simulink model "LaneKeeping"  (R2022b)
settings: Solver=ode8  StartTime=0.0  StopTime=inf  FixedStep=0.001  RelTol=1e-3
InitFcn:
  | start = 1
StopFcn:
  | start = 0
model workspace (MAT data in the model file):
  SL_ROS_VariableLengthArrays_MaxSizes.CommonInfo.ArrayTruncateAction = 'EmitWarning'
  SL_ROS_VariableLengthArrays_MaxSizes.MsgTypeMap = containers.Map
  SL_ROS_VariableLengthArrays_MaxSizes.MsgTypeMap.serialization.keys = {'sensor_msgs/CompressedImage'}
  SL_ROS_VariableLengthArrays_MaxSizes.MsgTypeMap.serialization.values{1}(1).PropertyName = 'Data'
  SL_ROS_VariableLengthArrays_MaxSizes.MsgTypeMap.serialization.values{1}(1).DataType = 'uint8'
  SL_ROS_VariableLengthArrays_MaxSizes.MsgTypeMap.serialization.values{1}(1).MaxLength = 220631000
  SL_ROS_VariableLengthArrays_MaxSizes.MsgTypeMap.serialization.values{1}(2).PropertyName = 'Format'
  SL_ROS_VariableLengthArrays_MaxSizes.MsgTypeMap.serialization.values{1}(2).DataType = 'uint8'
  SL_ROS_VariableLengthArrays_MaxSizes.MsgTypeMap.serialization.values{1}(2).MaxLength = 128
  SL_ROS_VariableLengthArrays_MaxSizes.MsgTypeMap.serialization.uniformity = 0
  SL_ROS_VariableLengthArrays_MaxSizes.MsgTypeMap.serialization.keyType = 'char'
  SL_ROS_VariableLengthArrays_MaxSizes.MsgTypeMap.serialization.valueType = 'any'
undefined symbols (not defined in the file): gray, L, r, Rec, SDTV, VelLeft, VelRight
libraries: robotlib x6, visiontextngfix x6, simulink_extras x6, visionconversions x5, visiontransforms x4, dspstat3 x4, dspmtrx3 x4, visionfilter x2, matrix_library x2, visionanalysis x2, visionstatistics x2, slpidlib x1
settings Model: Creator=gaetano  LastModifiedBy=gaetano

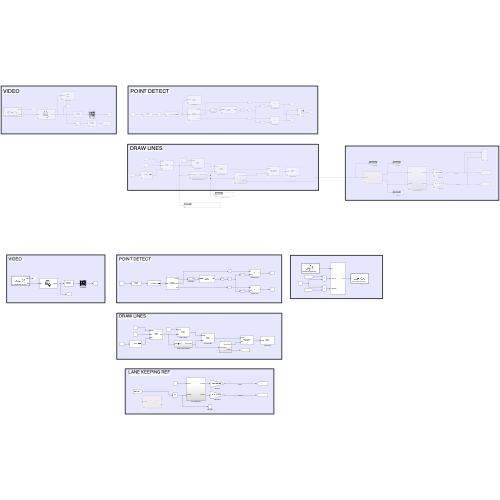
[thumbnail: Simulink's stored preview of the top-level diagram]
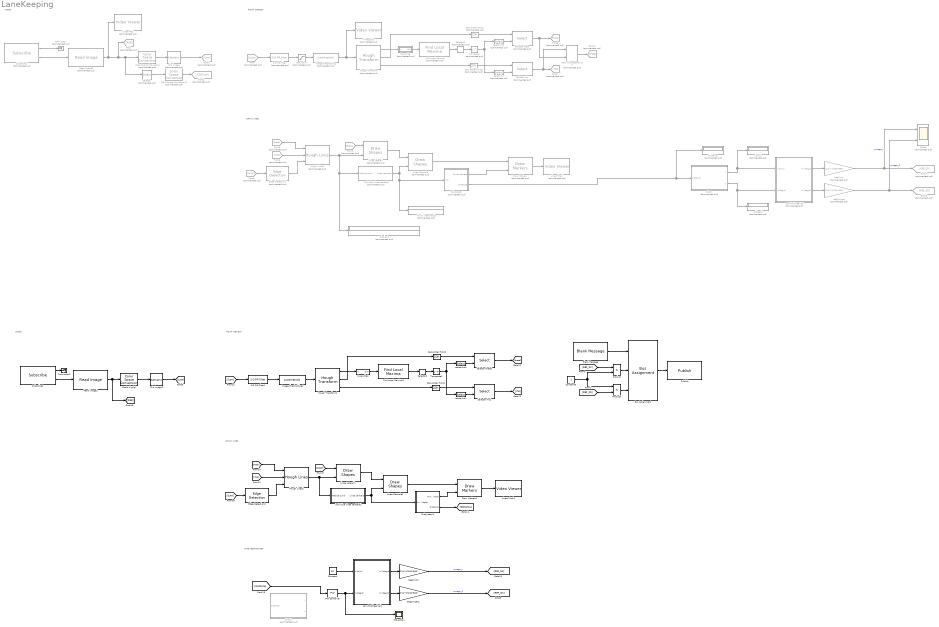
== system LaneKeeping ==
  note: VIDEO
  note: POINT DETECT
  note: DRAW LINES
  note: LANE KEEPING REF
  note: DRAW LINES
  note: POINT DETECT
  note: VIDEO
  2-D FIR Filter : visionfilter/2-D FIR Filter  Commented=on  separable=off  filtSrc=Specify via dialog  filterMtrx=[-1 0 1]  verticalFilter=[4 0]  horizontalFilter=[4 0]  outSize=Same as input port I  padType=Replicate  padSrc=Specify via dialog  padVal=0  method=Convolution  firstCoeffMode=Specify word length  firstCoeffWordLength=16  firstCoeffFracLength=14  firstCoeffSignedness=Signed  firstCoeffLastDataTypeStr=fixdt(1,16)  outputSignedness=Auto  accumLastDataTypeStr=Inherit: Same as product output  prodOutputMode=Binary point scaling  prodOutputWordLength=32  prodOutputFracLength=10  prodOutputLastDataTypeStr=fixdt([],32,10)  roundingMode=Floor  overflowMode=on  firstCoeffDataTypeStr=fixdt(1,16)  firstCoeffMin=[]  firstCoeffMax=[]  prodOutputDataTypeStr=fixdt([],32,10)  accumDataTypeStr=Inherit: Same as product output  outputMin=[]  outputMax=[]
  2-D FIR Filter1 : visionfilter/2-D FIR Filter  separable=off  filtSrc=Specify via dialog  filterMtrx=[-1 0 1]  verticalFilter=[4 0]  horizontalFilter=[4 0]  outSize=Same as input port I  padType=Replicate  padSrc=Specify via dialog  padVal=0  method=Convolution  firstCoeffMode=Specify word length  firstCoeffWordLength=16  firstCoeffFracLength=14  firstCoeffSignedness=Signed  firstCoeffLastDataTypeStr=fixdt(1,16)  outputSignedness=Auto  accumLastDataTypeStr=Inherit: Same as product output  prodOutputMode=Binary point scaling  prodOutputWordLength=32  prodOutputFracLength=10  prodOutputLastDataTypeStr=fixdt([],32,10)  roundingMode=Floor  overflowMode=on  firstCoeffDataTypeStr=fixdt(1,16)  firstCoeffMin=[]  firstCoeffMax=[]  prodOutputDataTypeStr=fixdt([],32,10)  accumDataTypeStr=Inherit: Same as product output  outputMin=[]  outputMax=[]
  Blank Message : robotlib/Blank Message  messageClass=Message  entityType=duckietown_msgs/WheelsCmdStamped  messageType=duckietown_msgs/WheelsCmdStamped  SampleTime=-1  legacyBusStruct=off
      settings: LibrarySourceBlock=roslib/ROS/Blank Message
  Bus Assignment : BusAssignment  AssignedSignals=VelLeft,VelRight
  Chart : Stateflow chart  Commented=on  TreatAsAtomicUnit=on
  Chart1 : Stateflow chart  Commented=on  TreatAsAtomicUnit=on
  Clip image : matrix_library/Submatrix  Commented=on  RowSpan=Range of rows  RowStartMode=Offset from middle  RowStartIndex=1  RowEndMode=Last  RowEndIndex=1  ColSpan=All columns  ColStartMode=First  ColStartIndex=1  ColEndMode=Last  ColEndIndex=1
  Clip image1 : matrix_library/Submatrix  RowSpan=Range of rows  RowStartMode=Offset from middle  RowStartIndex=15  RowEndMode=Last  RowEndIndex=1  ColSpan=All columns  ColStartMode=First  ColStartIndex=1  ColEndMode=Last  ColEndIndex=1
  Color Space Conversion : visionconversions/Color Space  Conversion  Commented=on  conversion=Obsolete  conversionActive=R'G'B' to intensity  wp_str=D65  rec=Rec. 601 (SDTV)  sys=1125/60/2:1  imagePorts=One multidimensional signal
  Color Space Conversion1 : visionconversions/Color Space  Conversion  Commented=on  conversion=Obsolete  conversionActive=R'G'B' to Y'CbCr  wp_str=D65  rec=Rec. 601 (SDTV)  sys=1125/60/2:1  imagePorts=One multidimensional signal
  Constant : Constant  Value=10
  Constant3 : Constant  OutDataTypeStr=single
  Display2 : Display  Commented=on
  Distanza : Display  Commented=on
  Draw Markers : visiontextngfix/Draw Markers  Commented=on  shape=X-mark  size=3  fill=off  fillClrSource=Specify via dialog  display=White  intensity=200  color=[250 0 0]  opacity=0.6  viewport=Entire image  antialiasing=off  inType=Obsolete  imagePorts=One multidimensional signal  roundingMode=Floor  overflowMode=off  memoryMode=Specify word length  memoryWordLength=16  memoryFracLength=15  prodOutputMode=Binary point scaling  prodOutputWordLength=32  prodOutputFracLength=14
  Draw Markers1 : visiontextngfix/Draw Markers  shape=X-mark  size=3  fill=off  fillClrSource=Specify via dialog  display=White  intensity=200  color=[250 0 0]  opacity=0.6  viewport=Entire image  antialiasing=off  inType=Obsolete  imagePorts=One multidimensional signal  roundingMode=Floor  overflowMode=off  memoryMode=Specify word length  memoryWordLength=16  memoryFracLength=15  prodOutputMode=Binary point scaling  prodOutputWordLength=32  prodOutputFracLength=14
  Edge Detection1 : visionanalysis/Edge Detection  Commented=on  method=Sobel  outputType=Binary image  userDefinedThreshold=off  thresholdSource=Input port  threshold=20  thresholdTuning=4  edgeThinning=off  threshold_canny=[0.25 0.60]  autoPercent=70  sigma=1  roundingMode=Floor  overflowMode=off  prodOutputMode=Binary point scaling  prodOutputWordLength=32  prodOutputFracLength=8
  Edge Detection2 : visionanalysis/Edge Detection  method=Sobel  outputType=Binary image  userDefinedThreshold=off  thresholdSource=Input port  threshold=20  thresholdTuning=4  edgeThinning=off  threshold_canny=[0.25 0.60]  autoPercent=70  sigma=1  roundingMode=Floor  overflowMode=off  prodOutputMode=Binary point scaling  prodOutputWordLength=32  prodOutputFracLength=8
  Find Local Maxima : visionstatistics/Find Local Maxima  Commented=on  num_peaks=2  nhood_size=[301 81]  src_thresh=Obsolete9b  src_thresh_inuse=Specify via dialog  threshold=1  inputIsHough=on  dt_peak=uint16  isOutVarDim=on  dt_count=uint16
  Find Local Maxima1 : visionstatistics/Find Local Maxima  num_peaks=2  nhood_size=[301 81]  src_thresh=Obsolete9b  src_thresh_inuse=Specify via dialog  threshold=1  inputIsHough=on  dt_peak=uint16  isOutVarDim=on  dt_count=uint16
  From : From  Commented=on  GotoTag=ILow
  From5 : From  Commented=on  GotoTag=theta
  From6 : From  Commented=on  GotoTag=rho
  From8 : From  Commented=on  GotoTag=ILow
  From9 : From  Commented=on  GotoTag=ILow
  Goto : Goto  Commented=on  GotoTag=RGB
  Goto1 : Goto  Commented=on  GotoTag=ILow
  Goto2 : Goto  Commented=on  GotoTag=YCbCrLow
  Goto3 : Goto  Commented=on  GotoTag=REF_DX
  Goto4 : Goto  Commented=on  GotoTag=REF_SX
  Goto6 : Goto  Commented=on  GotoTag=theta
  Goto7 : Goto  Commented=on  GotoTag=rho
  Goto8 : Goto  Commented=on  GotoTag=lines
  Hough Lines1 : visiontransforms/Hough Lines  Commented=on  sineCompMethod=Trigonometric function  thetaRes=pi/180  roundingMode=Nearest  overflowMode=on  firstCoeffMode=Specify word length  firstCoeffWordLength=16  prodOutputMode=Binary point scaling  prodOutputWordLength=32  prodOutputFracLength=16  firstCoeffFracLength=15
  Hough Lines2 : visiontransforms/Hough Lines  sineCompMethod=Trigonometric function  thetaRes=pi/180  roundingMode=Nearest  overflowMode=on  firstCoeffMode=Specify word length  firstCoeffWordLength=16  prodOutputMode=Binary point scaling  prodOutputWordLength=32  prodOutputFracLength=16  firstCoeffFracLength=15
  Hough Transform : visiontransforms/Hough Transform  Commented=on  theta_res=pi/180  rho_res=1  out_theta_rho=on  outdtmode=single  roundingMode=Nearest  overflowMode=on  firstCoeffMode=Binary point scaling  firstCoeffWordLength=16  firstCoeffFracLength=14  secondCoeffMode=Binary point scaling  secondCoeffWordLength=32  secondCoeffFracLength=16  prodOutputMode=Binary point scaling  prodOutputWordLength=32  prodOutputFracLength=20  accumMode=Binary point scaling  accumWordLength=32  accumFracLength=20  outputMode=Binary point scaling  outputWordLength=16  outputFracLength=0  memoryMode=Binary point scaling  memoryWordLength=32  memoryFracLength=16
  Hough Transform1 : visiontransforms/Hough Transform  theta_res=pi/180  rho_res=1  out_theta_rho=on  outdtmode=single  roundingMode=Nearest  overflowMode=on  firstCoeffMode=Binary point scaling  firstCoeffWordLength=16  firstCoeffFracLength=14  secondCoeffMode=Binary point scaling  secondCoeffWordLength=32  secondCoeffFracLength=16  prodOutputMode=Binary point scaling  prodOutputWordLength=32  prodOutputFracLength=20  accumMode=Binary point scaling  accumWordLength=32  accumFracLength=20  outputMode=Binary point scaling  outputWordLength=16  outputFracLength=0  memoryMode=Binary point scaling  memoryWordLength=32  memoryFracLength=16
  Image thresholding : visionconversions/Autothreshold  Commented=on  operator=>  threshOut=off  effMetricOut=off  userDefinedRange=off  umin=50  umax=255  outOfRngOpt=Ignore  scaleThreshold=off  scaleFactor=1  roundingMode=Floor  overflowMode=off  P1Mode=Specify word length  P1WordLength=32  P1FracLength=30  P2Mode=Specify word length  P2WordLength=32  P2FracLength=22  P3Mode=Specify word length  P3WordLength=32  P3FracLength=14  P4Mode=Binary point scaling  P4WordLength=32  P4FracLength=15  Q1Mode=Specify word length  Q1WordLength=32  Q1FracLength=16  EMMode=Specify word length  EMWordLength=16  EMFracLength=14
  Image thresholding1 : visionconversions/Autothreshold  operator=>  threshOut=off  effMetricOut=off  userDefinedRange=off  umin=50  umax=255  outOfRngOpt=Ignore  scaleThreshold=off  scaleFactor=1  roundingMode=Floor  overflowMode=off  P1Mode=Specify word length  P1WordLength=32  P1FracLength=30  P2Mode=Specify word length  P2WordLength=32  P2FracLength=22  P3Mode=Specify word length  P3WordLength=32  P3FracLength=14  P4Mode=Binary point scaling  P4WordLength=32  P4FracLength=15  Q1Mode=Specify word length  Q1WordLength=32  Q1FracLength=16  EMMode=Specify word length  EMWordLength=16  EMFracLength=14
  Individua linea centrale : Subsystem  Commented=on
  Individua linea centrale1 : Subsystem
  Linea Centrale : visiontextngfix/Draw Shapes  Commented=on  shape=Lines  fill=off  lineWidth=2  fillClrSource=Specify via dialog  display=White  intensity=200  color=[200 255 100]  opacity=0.6  viewport=Entire image  antialiasing=off  inType=Obsolete  imagePorts=One multidimensional signal  roundingMode=Floor  overflowMode=off  memoryMode=Specify word length  memoryWordLength=16  prodOutputMode=Binary point scaling  prodOutputWordLength=32  prodOutputFracLength=14  memoryFracLength=15
  Linea Centrale1 : visiontextngfix/Draw Shapes  shape=Lines  fill=off  lineWidth=2  fillClrSource=Specify via dialog  display=White  intensity=200  color=[200 255 100]  opacity=0.6  viewport=Entire image  antialiasing=off  inType=Obsolete  imagePorts=One multidimensional signal  roundingMode=Floor  overflowMode=off  memoryMode=Specify word length  memoryWordLength=16  prodOutputMode=Binary point scaling  prodOutputWordLength=32  prodOutputFracLength=14  memoryFracLength=15
  Linee Finali : VideoViewer  Commented=on  colormapValue=gray(256)  FigPos=[831 826 610 698]
  Linee Finali1 : VideoViewer  colormapValue=gray(256)  FigPos=[342 823 793 695]
  Linee Laterali : visiontextngfix/Draw Shapes  Commented=on  shape=Lines  fill=off  lineWidth=2  fillClrSource=Specify via dialog  display=White  intensity=200  color=[200 255 100]  opacity=0.6  viewport=Entire image  antialiasing=off  inType=Obsolete  imagePorts=One multidimensional signal  roundingMode=Floor  overflowMode=off  memoryMode=Specify word length  memoryWordLength=16  prodOutputMode=Binary point scaling  prodOutputWordLength=32  prodOutputFracLength=14  memoryFracLength=15
  Linee Laterali1 : visiontextngfix/Draw Shapes  shape=Lines  fill=off  lineWidth=2  fillClrSource=Specify via dialog  display=White  intensity=200  color=[200 255 100]  opacity=0.6  viewport=Entire image  antialiasing=off  inType=Obsolete  imagePorts=One multidimensional signal  roundingMode=Floor  overflowMode=off  memoryMode=Specify word length  memoryWordLength=16  prodOutputMode=Binary point scaling  prodOutputWordLength=32  prodOutputFracLength=14  memoryFracLength=15
  Matrix Concatenation3 : Concatenate  Commented=on  Mode=Multidimensional array
  Overwrite : Subsystem  Commented=on
  Overwrite1 : Subsystem
  PID Controller : slpidlib/PID Controller  Controller=P  Form=Parallel  TimeDomain=Continuous-time  UseExternalTs=off  SampleTime=-1  IntegratorMethod=Forward Euler  FilterMethod=Forward Euler  ControllerParametersSource=internal  P=0.28  I=1  UseKiTs=off  D=0  N=100  UseFilter=on  TunerSelectOption=Transfer Function Based (PID Tuner App)  InitialConditionSource=internal  InitialConditionForIntegrator=0  InitialConditionForFilter=0  DifferentiatorICPrevScaledInput=0  ExternalReset=none  TrackingMode=off  Kt=1  LimitOutput=off  SatLimitsSource=internal  UpperSaturationLimit=40  LowerSaturationLimit=-40  LinearizeAsGain=off  AntiWindupMode=none  Kb=1  LimitIntegrator=off  UpperIntegratorSaturationLimit=inf  LowerIntegratorSaturationLimit=-inf  PGainOutDataTypeStr=double  PProdOutDataTypeStr=double  POutMin=[]  POutMax=[]  IOutMin=[]  IOutMax=[]  DOutMin=[]  DOutMax=[]  NOutMin=[]  NOutMax=[]  SumOutMin=[]  SumOutMax=[]  SaturationOutMin=[]  SaturationOutMax=[]  PParamMin=[]  PParamMax=[]  IParamMin=[]  IParamMax=[]  DParamMin=[]  DParamMax=[]  NParamMin=[]  NParamMax=[]  KbParamMin=[]  KbParamMax=[]  KtParamMin=[]  KtParamMax=[]  KbOutMin=[]  KbOutMax=[]  KtOutMin=[]  KtOutMax=[]  IntegratorOutMin=[]  IntegratorOutMax=[]  FilterOutMin=[]  FilterOutMax=[]  SumI1OutMin=[]  SumI1OutMax=[]  SumI2OutMin=[]  SumI2OutMax=[]  SumI3OutMin=[]  SumI3OutMax=[]  SumI4OutMin=[]  SumI4OutMax=[]  SumDOutMin=[]  SumDOutMax=[]  DifferentiatorOutMin=[]  DifferentiatorOutMax=[]  FilterDiffOutCoefMin=[]  FilterDiffOutCoefMax=[]  ReciprocalOutMin=[]  ReciprocalOutMax=[]  SumDenOutMin=[]  SumDenOutMax=[]  SumNumOutMin=[]  SumNumOutMax=[]  DivideOutMin=[]  DivideOutMax=[]  UdiffTsProdOutMin=[]  UdiffTsProdOutMax=[]  NTsProdOutMin=[]  NTsProdOutMax=[]  UintegralTsProdOutMin=[]  UintegralTsProdOutMax=[]  UngainTsProdOutMin=[]  UngainTsProdOutMax=[]  ClampingZeroOutDataTypeStr=Inherit: Inherit via back propagation  ClampingZeroOutMin=[]  ClampingZeroOutMax=[]  FilterDenConstantOutDataTypeStr=Inherit: Inherit via back propagation  FilterDenConstantOutMin=[]  FilterDenConstantOutMax=[]  PCopyOutDataTypeStr=Inherit: Inherit via back propagation  PCopyOutMin=[]  PCopyOutMax=[]  NCopyOutDataTypeStr=Inherit: Inherit via back propagation  NCopyOutMin=[]  NCopyOutMax=[]  IntegratorContinuousStateAttributes=''  IntegratorStateMustResolveToSignalObject=off  IntegratorRTWStateStorageClass=Auto  FilterContinuousStateAttributes=''  FilterStateMustResolveToSignalObject=off  FilterRTWStateStorageClass=Auto  ParallelPVariant=InternalParameters  IdealPVariant=Disabled  IVariant=Disabled  DVariant=Disabled  IntegratorVariant=Disabled  SatVariant=Disabled  AWVariant=Disabled  PCopyVariant=Disabled  TRVariant=Disabled  FdbkBlocksVariant=Forward  IdealPFdbkVariant=Disabled  SatFdbkVariant=Disabled  DerivativeFilterVariant=Disabled  NVariant=Disabled  NCopyVariant=Disabled_SignalSpec  FilterICVariant=Disabled  IntegratorICVariant=Disabled  ExternalResetVariant=Disabled  TRSumVariant=Passthrough  SumFdbkVariant=Disabled  SumVariant=Passthrough_P  TsampFilterVariant=InternalTs  TsampNgainVariant=Passthrough  TsampIntegralVariant=Disabled_SignalSpec  ExternalSaturationOutDataTypeStr=Inherit: Same as second input
  PID_action : Scope
  Product : Product  OutDataTypeStr=single
  Product1 : Product  OutDataTypeStr=single
  Publish : robotlib/Publish  topicSource=Select from ROS network  topic=/vic9osimhen/wheels_driver_node/wheels_cmd  messageType=duckietown_msgs/WheelsCmdStamped  legacyBusStruct=off  messageQueueLength=1
      settings: LibrarySourceBlock=roslib/ROS/Publish
  Punti linea media : Display  Commented=on
  Read Image1 : robotlib/Read Image  Commented=on  MaximumImageSize=[480,640]  ImageEncoding=rgb8  ShowAlphaOutput=off  ShowErrorCodeOutput=off  VariableSizeOutputs=off
      settings: LibrarySourceBlock=roslib/ROS/Read Image
  Read Image2 : robotlib/Read Image  MaximumImageSize=[480,640]  ImageEncoding=rgb8  ShowAlphaOutput=off  ShowErrorCodeOutput=off  VariableSizeOutputs=off
      settings: LibrarySourceBlock=roslib/ROS/Read Image
  Saturation : Saturate  Commented=on  UpperLimit=1  LowerLimit=0
  Scala di grigi : visionconversions/Color Space  Conversion  conversion=Obsolete  conversionActive=R'G'B' to intensity  wp_str=D65  rec=Rec. 601 (SDTV)  sys=1125/60/2:1  imagePorts=One multidimensional signal
  Scope : Scope  Commented=on  NumInputPorts=2
  Selector : Selector  Commented=on  NumberOfDimensions=3  InputPortWidth=3  IndexOptions=Index vector (dialog),Select all,Select all  Indices=(640/2+1):480,1,2  OutputSizes=1,1,1
  Selector rho : Selector  Commented=on  NumberOfDimensions=2  InputPortWidth=3  IndexOptions=Select all,Index vector (port)  Indices=1,2  OutputSizes=1,1
  Selector rho1 : Selector  NumberOfDimensions=2  InputPortWidth=3  IndexOptions=Select all,Index vector (port)  Indices=1,2  OutputSizes=1,1
  Selector theta : Selector  Commented=on  NumberOfDimensions=2  InputPortWidth=3  IndexOptions=Select all,Index vector (port)  Indices=1,2  OutputSizes=1,1
  Selector theta1 : Selector  NumberOfDimensions=2  InputPortWidth=3  IndexOptions=Select all,Index vector (port)  Indices=1,2  OutputSizes=1,1
  Selector1 : Selector  Commented=on  NumberOfDimensions=2  InputPortWidth=3  IndexOptions=Select all,Index vector (dialog)  Indices=[2 1],[2 1]  OutputSizes=1,1
  Selector2 : Selector  NumberOfDimensions=2  InputPortWidth=3  IndexOptions=Select all,Index vector (dialog)  Indices=[2 1],[2 1]  OutputSizes=1,1
  Subscribe1 : robotlib/Subscribe  Commented=on  topicSource=Select from ROS network  topic=/vic9osimhen/camera_node/image/compressed  messageType=sensor_msgs/CompressedImage  SampleTime=-1  legacyBusStruct=off  messageQueueLength=1
      settings: LibrarySourceBlock=roslib/ROS/Subscribe
  Subscribe2 : robotlib/Subscribe  topicSource=Select from ROS network  topic=/vic9osimhen/camera_node/image/compressed  messageType=sensor_msgs/CompressedImage  SampleTime=-1  legacyBusStruct=off  messageQueueLength=1
      settings: LibrarySourceBlock=roslib/ROS/Subscribe
  Subsystem : Subsystem  Commented=on
  Subsystem1 : Subsystem
  Terminator : Terminator  Commented=on
  Terminator1 : Terminator
  Threshold : VideoViewer  Commented=on  colormapValue=gray(256)  FigPos=[280 584 557 295]
  Transpose : Math  Commented=on  Operator=transpose  SignedPower=on
  Transpose1 : Math  Operator=transpose  SignedPower=on
  Video ROS : VideoViewer  Commented=on  colormapValue=gray(256)  FigPos=[1 826 566 334]
  Zero-Order Hold1 : ZeroOrderHold  Commented=on  SampleTime=-1
  Zero-Order Hold2 : ZeroOrderHold  SampleTime=-1
  Zero-Order Hold3 : ZeroOrderHold  Commented=on  SampleTime=-1
  Zero-Order Hold4 : ZeroOrderHold  SampleTime=-1
  convToWheelVel : Subsystem  Commented=on
  convToWheelVel1 : Subsystem
  deg2m/s : Gain  Commented=on  Gain=(2*pi*r)/(100*360)
  deg2m/s1 : Gain  Gain=(2*pi*r)/(100*360)
  deg2m/sec : Gain  Commented=on  Gain=(2*pi*r)/(100*360)
  deg2m/sec1 : Gain  Gain=(2*pi*r)/(100*360)
  select rho : Selector  Commented=on  NumberOfDimensions=2  InputPortWidth=3  IndexOptions=Index vector (dialog),Select all  Indices=1,-1  OutputSizes=1
  select rho1 : Selector  NumberOfDimensions=2  InputPortWidth=3  IndexOptions=Index vector (dialog),Select all  Indices=1,-1  OutputSizes=1
  select rho2 : Selector  NumberOfDimensions=2  InputPortWidth=3  IndexOptions=Index vector (dialog),Select all  Indices=2,-1  OutputSizes=1
  select rho3 : Selector  Commented=on  NumberOfDimensions=2  InputPortWidth=3  IndexOptions=Index vector (dialog),Select all  Indices=2,-1  OutputSizes=1
  v(cm/s) : Display  Commented=on
  w(deg/s) : Display  Commented=on
  wires:
  Color Space Conversion/1 -> Clip image/1
  Color Space Conversion1/1 -> Goto2/1
  Clip image/1 -> Goto1/1
  Selector/1 -> Color Space Conversion1/1
  From/1 -> 2-D FIR Filter/1
  Image thresholding/1 -> Hough Transform/1, Threshold/1
  2-D FIR Filter/1 -> Saturation/1
  Saturation/1 -> Image thresholding/1
  Matrix Concatenation3/1 -> Goto8/1
  Hough Transform/1 -> Overwrite/1(In)
  Transpose/1 -> select rho/1, select rho3/1
  Selector1/1 -> Transpose/1
  Find Local Maxima/1 -> Selector1/1
  Hough Transform/3 -> Zero-Order Hold3/1
  select rho/1 -> Selector rho/2
  Zero-Order Hold3/1 -> Selector rho/1
  Hough Transform/2 -> Zero-Order Hold1/1
  select rho3/1 -> Selector theta/2
  Zero-Order Hold1/1 -> Selector theta/1
  Selector rho/1 -> Goto7/1, Matrix Concatenation3/1
  Selector theta/1 -> Goto6/1, Matrix Concatenation3/2
  Overwrite/1(Out) -> Find Local Maxima/1
  From5/1 -> Hough Lines1/1
  Edge Detection1/1 -> Hough Lines1/3
  From6/1 -> Hough Lines1/2
  Subscribe1/1 -> Terminator/1
  Subscribe1/2 -> Read Image1/1
  From8/1 -> Edge Detection1/1
  From9/1 -> Linee Laterali/1
  Linee Laterali/1 -> Linea Centrale/1
  Linea Centrale/1 -> Draw Markers/1
  Hough Lines1/1 -> Display2/1, Individua linea centrale/1(Matrice punti), Linee Laterali/2
  Individua linea centrale/1(Linea centrale) -> Linea Centrale/2, Punti linea media/1, Subsystem/1(In1)
  Draw Markers/1 -> Linee Finali/1
  Subsystem/1(Punto camera) -> Draw Markers/2
  Subsystem/2(Distanza) -> Distanza/1, Chart/1(distanza)
  Chart/1(v) -> v(cm/s)/1, convToWheelVel/1(v(cm/s))
  Chart/2(w) -> convToWheelVel/2(w(deg/s)), w(deg/s)/1
  convToWheelVel/1(wl (deg/s)) -> deg2m/s/1
  deg2m/sec/1 -> Goto3/1, Scope/2  "omega_R"
  deg2m/s/1 -> Goto4/1, Scope/1  "omega_L"
  convToWheelVel/2(wr (deg/s)) -> deg2m/sec/1
  Bus Assignment/1 -> Publish/1
  Blank Message/1 -> Bus Assignment/1
  Product/1 -> Bus Assignment/2
  Product1/1 -> Bus Assignment/3
  [REF_SX] -> Product/1
  [REF_DX] -> Product1/2
  Constant3/1 -> Product1/1, Product/2
  Read Image1/1 -> Color Space Conversion/1, Selector/1, Goto/1, Video ROS/1
  select rho1/1 -> Selector rho1/2
  [ILow] -> 2-D FIR Filter1/1
  PID Controller/1 -> PID_action/1, convToWheelVel1/2(w(deg/s))
  Draw Markers1/1 -> Linee Finali1/1
  Image thresholding1/1 -> Hough Transform1/1
  Subsystem1/1(Punto camera) -> Draw Markers1/2
  Transpose1/1 -> select rho1/1, select rho2/1
  Zero-Order Hold4/1 -> Selector rho1/1
  Overwrite1/1(Out) -> Find Local Maxima1/1
  Hough Lines2/1 -> Individua linea centrale1/1(Matrice punti), Linee Laterali1/2
  Individua linea centrale1/1(Linea centrale) -> Subsystem1/1(Linea centrale), Linea Centrale1/2
  Constant/1 -> convToWheelVel1/1(v(cm/s))
  Clip image1/1 -> [ILow]
  2-D FIR Filter1/1 -> Image thresholding1/1
  [theta] -> Hough Lines2/1
  Subscribe2/1 -> Terminator1/1
  Edge Detection2/1 -> Hough Lines2/3
  Linea Centrale1/1 -> Draw Markers1/1
  convToWheelVel1/2(wr (deg/s)) -> deg2m/sec1/1
  deg2m/sec1/1 -> [REF_DX]  "omega_R"
  Selector2/1 -> Transpose1/1
  Subscribe2/2 -> Read Image2/1
  deg2m/s1/1 -> [REF_SX]  "omega_L"
  convToWheelVel1/1(wl (deg/s)) -> deg2m/s1/1
  Hough Transform1/2 -> Zero-Order Hold2/1
  Hough Transform1/3 -> Zero-Order Hold4/1
  Zero-Order Hold2/1 -> Selector theta1/1
  Scala di grigi/1 -> Clip image1/1
  select rho2/1 -> Selector theta1/2
  Hough Transform1/1 -> Overwrite1/1(In)
  [ILow] -> Edge Detection2/1
  Selector rho1/1 -> [rho]
  Subsystem1/2(Distanza) -> [Distanza]
  [Distanza] -> PID Controller/1
  Find Local Maxima1/1 -> Selector2/1
  Read Image2/1 -> [RGB], Scala di grigi/1
  [rho] -> Hough Lines2/2
  Selector theta1/1 -> [theta]
  Linee Laterali1/1 -> Linea Centrale1/1
  [ILow] -> Linee Laterali1/1

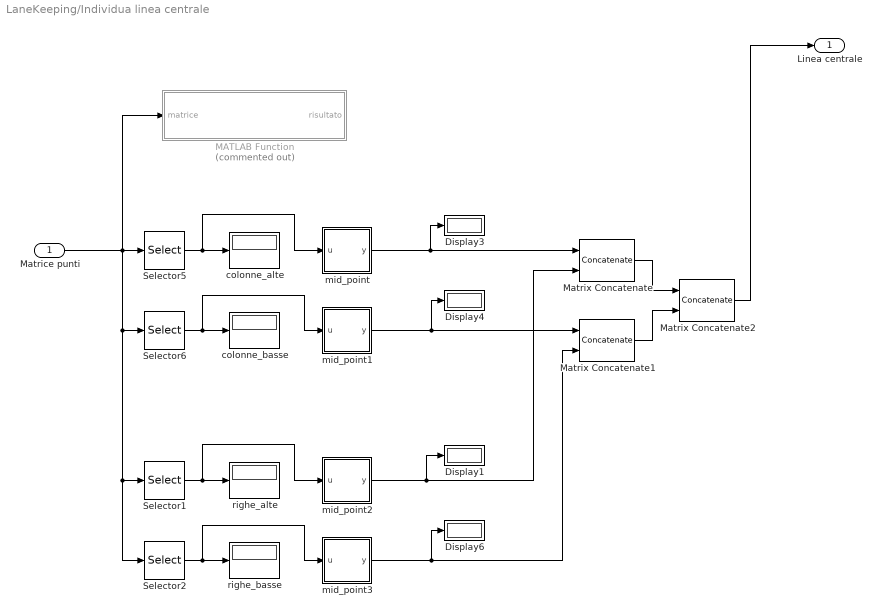
== system LaneKeeping/Individua linea centrale ==
  Matrice punti : Inport
  Display{1,3..4,6} (4 alike) : Display
  MATLAB Function : MATLAB Function  Commented=on  TreatAsAtomicUnit=on
  Matrix Concatenate : Concatenate  Mode=Multidimensional array
  Matrix Concatenate1 : Concatenate  Mode=Multidimensional array
  Matrix Concatenate2 : Concatenate  Mode=Multidimensional array
  Selector1 : Selector  NumberOfDimensions=2  InputPortWidth=3  IndexOptions=Index vector (dialog),Index vector (dialog)  Indices=[1 2],[2]  OutputSizes=1,1
  Selector2 : Selector  NumberOfDimensions=2  InputPortWidth=3  IndexOptions=Index vector (dialog),Index vector (dialog)  Indices=[1 2],[4]  OutputSizes=1,1
  Selector5 : Selector  NumberOfDimensions=2  InputPortWidth=3  IndexOptions=Index vector (dialog),Index vector (dialog)  Indices=[1 2],[1]  OutputSizes=1,1
  Selector6 : Selector  NumberOfDimensions=2  InputPortWidth=3  IndexOptions=Index vector (dialog),Index vector (dialog)  Indices=[1 2],[3]  OutputSizes=1,1
  colonne_alte : Display
  colonne_basse : Display
  mid_point : MATLAB Function  TreatAsAtomicUnit=on
  mid_point1 : MATLAB Function  TreatAsAtomicUnit=on
  mid_point2 : MATLAB Function  TreatAsAtomicUnit=on
  mid_point3 : MATLAB Function  TreatAsAtomicUnit=on
  righe_alte : Display
  righe_basse : Display
  Linea centrale : Outport
  wires:
  Matrix Concatenate/1 -> Matrix Concatenate2/1
  mid_point1/1(y) -> Matrix Concatenate1/1, Display4/1
  Selector5/1 -> mid_point/1(u), colonne_alte/1
  mid_point/1(y) -> Display3/1, Matrix Concatenate/1
  Matrix Concatenate1/1 -> Matrix Concatenate2/2
  Matrice punti/1 -> Selector2/1, Selector1/1, Selector6/1, MATLAB Function/1(matrice), Selector5/1
  Matrix Concatenate2/1 -> Linea centrale/1
  Selector6/1 -> colonne_basse/1, mid_point1/1(u)
  mid_point2/1(y) -> Matrix Concatenate/2, Display1/1
  mid_point3/1(y) -> Display6/1, Matrix Concatenate1/2
  Selector2/1 -> righe_basse/1, mid_point3/1(u)
  Selector1/1 -> mid_point2/1(u), righe_alte/1

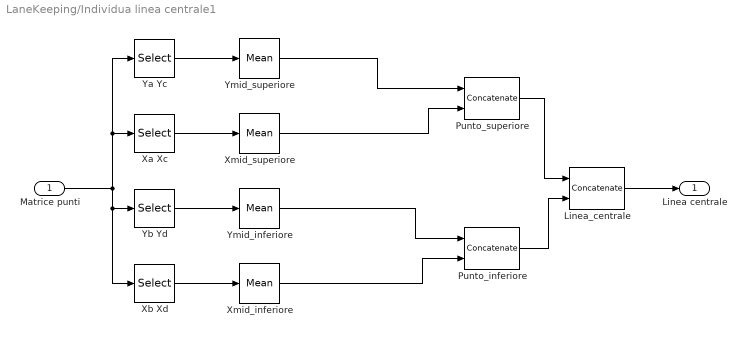
== system LaneKeeping/Individua linea centrale1 ==
  Matrice punti : Inport
  Linea_centrale : Concatenate  Mode=Multidimensional array
  Punto_inferiore : Concatenate  Mode=Multidimensional array
  Punto_superiore : Concatenate  Mode=Multidimensional array
  Xa Xc : Selector  NumberOfDimensions=2  InputPortWidth=3  IndexOptions=Index vector (dialog),Index vector (dialog)  Indices=[1 2],[2]  OutputSizes=1,1
  Xb Xd : Selector  NumberOfDimensions=2  InputPortWidth=3  IndexOptions=Index vector (dialog),Index vector (dialog)  Indices=[1 2],[4]  OutputSizes=1,1
  Xmid_inferiore : dspstat3/Mean  run=off  InputProcessing=Columns as channels (frame based)  reset_popup=None  directionMode=Each column  dimension=1  roiEnable=off  roiType=Rectangles  roiPortion=Entire ROI  roiOutput=Individual statistics for each ROI  roiFlag=off  roundingMode=Floor  overflowMode=off  outputDataTypeStr=Inherit: Same as accumulator  outputMin=[]  outputMax=[]  outputLastDataTypeStr=Inherit: Same as accumulator
  Xmid_superiore : dspstat3/Mean  run=off  InputProcessing=Columns as channels (frame based)  reset_popup=None  directionMode=Each column  dimension=1  roiEnable=off  roiType=Rectangles  roiPortion=Entire ROI  roiOutput=Individual statistics for each ROI  roiFlag=off  roundingMode=Floor  overflowMode=off  outputDataTypeStr=Inherit: Same as accumulator  outputMin=[]  outputMax=[]  outputLastDataTypeStr=Inherit: Same as accumulator
  Ya Yc : Selector  NumberOfDimensions=2  InputPortWidth=3  IndexOptions=Index vector (dialog),Index vector (dialog)  Indices=[1 2],[1]  OutputSizes=1,1
  Yb Yd : Selector  NumberOfDimensions=2  InputPortWidth=3  IndexOptions=Index vector (dialog),Index vector (dialog)  Indices=[1 2],[3]  OutputSizes=1,1
  Ymid_inferiore : dspstat3/Mean  run=off  InputProcessing=Columns as channels (frame based)  reset_popup=None  directionMode=Each column  dimension=1  roiEnable=off  roiType=Rectangles  roiPortion=Entire ROI  roiOutput=Individual statistics for each ROI  roiFlag=off  roundingMode=Floor  overflowMode=off  outputDataTypeStr=Inherit: Same as accumulator  outputMin=[]  outputMax=[]  outputLastDataTypeStr=Inherit: Same as accumulator
  Ymid_superiore : dspstat3/Mean  run=off  InputProcessing=Columns as channels (frame based)  reset_popup=None  directionMode=Each column  dimension=1  roiEnable=off  roiType=Rectangles  roiPortion=Entire ROI  roiOutput=Individual statistics for each ROI  roiFlag=off  roundingMode=Floor  overflowMode=off  outputDataTypeStr=Inherit: Same as accumulator  outputMin=[]  outputMax=[]  outputLastDataTypeStr=Inherit: Same as accumulator
  Linea centrale : Outport
  wires:
  Punto_superiore/1 -> Linea_centrale/1
  Ymid_inferiore/1 -> Punto_inferiore/1
  Ya Yc/1 -> Ymid_superiore/1
  Ymid_superiore/1 -> Punto_superiore/1
  Punto_inferiore/1 -> Linea_centrale/2
  Matrice punti/1 -> Xb Xd/1, Yb Yd/1, Xa Xc/1, Ya Yc/1
  Linea_centrale/1 -> Linea centrale/1
  Yb Yd/1 -> Ymid_inferiore/1
  Xmid_superiore/1 -> Punto_superiore/2
  Xmid_inferiore/1 -> Punto_inferiore/2
  Xb Xd/1 -> Xmid_inferiore/1
  Xa Xc/1 -> Xmid_superiore/1

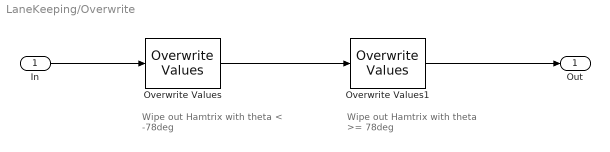
== system LaneKeeping/Overwrite ==
  note: Wipe out Hamtrix with
      | theta >=  78deg
  note: Wipe out Hamtrix with
      | theta <  -78deg
  In : Inport
  Overwrite Values : dspmtrx3/Overwrite Values  OverWriteDiag=Submatrix  valFrom2ndIP=Specify via dialog  ConstValue=0  RowSpan=All rows  RowStartMode=First  RowStartIndex=1  RowEndMode=Last  RowEndIndex=1  ColSpan=Range of columns  ColStartMode=First  ColStartIndex=1  ColEndMode=Index  ColEndIndex=12  DiagSpan=Range of elements  DiagStartMode=Index  DiagStartIndex=2  DiagEndMode=Index  DiagEndIndex=4
  Overwrite Values1 : dspmtrx3/Overwrite Values  OverWriteDiag=Submatrix  valFrom2ndIP=Specify via dialog  ConstValue=0  RowSpan=All rows  RowStartMode=First  RowStartIndex=1  RowEndMode=Last  RowEndIndex=1  ColSpan=Range of columns  ColStartMode=Offset from last  ColStartIndex=12  ColEndMode=Last  ColEndIndex=15  DiagSpan=Range of elements  DiagStartMode=Index  DiagStartIndex=2  DiagEndMode=Index  DiagEndIndex=4
  Out : Outport
  wires:
  Overwrite Values/1 -> Overwrite Values1/1
  In/1 -> Overwrite Values/1
  Overwrite Values1/1 -> Out/1

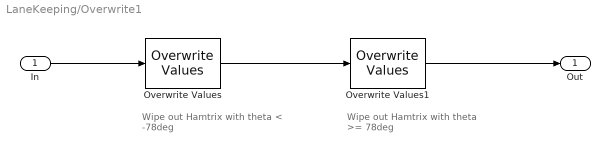
== system LaneKeeping/Overwrite1 ==
  note: Wipe out Hamtrix with
      | theta >=  78deg
  note: Wipe out Hamtrix with
      | theta <  -78deg
  In : Inport
  Overwrite Values : dspmtrx3/Overwrite Values  OverWriteDiag=Submatrix  valFrom2ndIP=Specify via dialog  ConstValue=0  RowSpan=All rows  RowStartMode=First  RowStartIndex=1  RowEndMode=Last  RowEndIndex=1  ColSpan=Range of columns  ColStartMode=First  ColStartIndex=1  ColEndMode=Index  ColEndIndex=12  DiagSpan=Range of elements  DiagStartMode=Index  DiagStartIndex=2  DiagEndMode=Index  DiagEndIndex=4
  Overwrite Values1 : dspmtrx3/Overwrite Values  OverWriteDiag=Submatrix  valFrom2ndIP=Specify via dialog  ConstValue=0  RowSpan=All rows  RowStartMode=First  RowStartIndex=1  RowEndMode=Last  RowEndIndex=1  ColSpan=Range of columns  ColStartMode=Offset from last  ColStartIndex=12  ColEndMode=Last  ColEndIndex=15  DiagSpan=Range of elements  DiagStartMode=Index  DiagStartIndex=2  DiagEndMode=Index  DiagEndIndex=4
  Out : Outport
  wires:
  Overwrite Values/1 -> Overwrite Values1/1
  In/1 -> Overwrite Values/1
  Overwrite Values1/1 -> Out/1

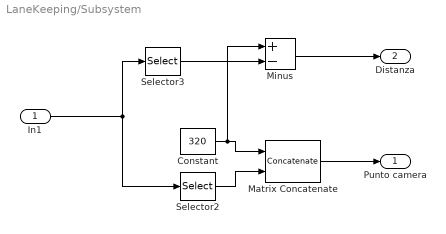
== system LaneKeeping/Subsystem ==
  In1 : Inport
  Constant : Constant  Value=320  OutDataTypeStr=int32
  Matrix Concatenate : Concatenate  Mode=Multidimensional array
  Minus : Sum  Inputs=+-
  Selector2 : Selector  InputPortWidth=4  IndexOptions=Index vector (dialog)  Indices=[4]  OutputSizes=1
  Selector3 : Selector  InputPortWidth=4  IndexOptions=Index vector (dialog)  Indices=[3]  OutputSizes=1
  Punto camera : Outport
  Distanza : Outport  Port=2
  wires:
  Minus/1 -> Distanza/1
  Constant/1 -> Minus/1, Matrix Concatenate/1
  In1/1 -> Selector3/1, Selector2/1
  Matrix Concatenate/1 -> Punto camera/1
  Selector2/1 -> Matrix Concatenate/2
  Selector3/1 -> Minus/2

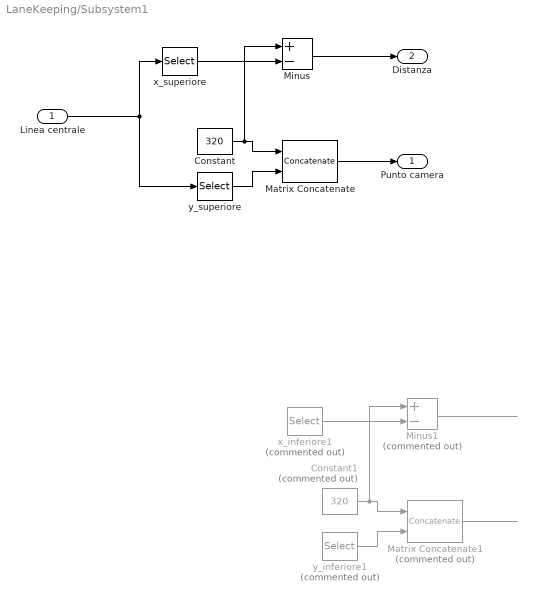
== system LaneKeeping/Subsystem1 ==
  Linea centrale : Inport
  Constant : Constant  Value=320  OutDataTypeStr=int32
  Constant1 : Constant  Commented=on  Value=320  OutDataTypeStr=int32
  Matrix Concatenate : Concatenate  Mode=Multidimensional array
  Matrix Concatenate1 : Concatenate  Commented=on  Mode=Multidimensional array
  Minus : Sum  Inputs=+-
  Minus1 : Sum  Commented=on  Inputs=+-
  x_inferiore1 : Selector  Commented=on  InputPortWidth=4  IndexOptions=Index vector (dialog)  Indices=[3]  OutputSizes=1
  x_superiore : Selector  InputPortWidth=4  IndexOptions=Index vector (dialog)  Indices=[1]  OutputSizes=1
  y_inferiore1 : Selector  Commented=on  InputPortWidth=4  IndexOptions=Index vector (dialog)  Indices=[4]  OutputSizes=1
  y_superiore : Selector  InputPortWidth=4  IndexOptions=Index vector (dialog)  Indices=[2]  OutputSizes=1
  Punto camera : Outport
  Distanza : Outport  Port=2
  wires:
  Minus/1 -> Distanza/1
  Constant/1 -> Minus/1, Matrix Concatenate/1
  Linea centrale/1 -> x_superiore/1, y_superiore/1
  Matrix Concatenate/1 -> Punto camera/1
  y_superiore/1 -> Matrix Concatenate/2
  x_superiore/1 -> Minus/2
  Matrix Concatenate1/1 -> ?
  y_inferiore1/1 -> Matrix Concatenate1/2
  ? -> x_inferiore1/1, y_inferiore1/1
  x_inferiore1/1 -> Minus1/2
  Minus1/1 -> ?
  Constant1/1 -> Minus1/1, Matrix Concatenate1/1

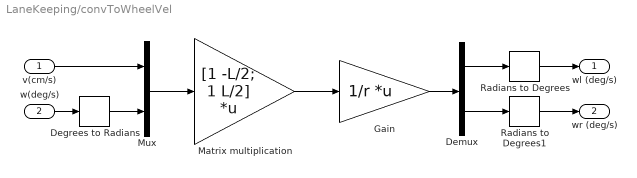
== system LaneKeeping/convToWheelVel ==
  v(cm/s) : Inport
  w(deg/s) : Inport  Port=2
  " Gain" : Gain  Gain=1/r  Multiplication=Matrix(K*u)
  Degrees to Radians : simulink_extras/Transformations/Degrees to Radians
  Demux : Demux  Outputs=2
  Matrix multiplication : Gain  Gain=[1 -L/2; 1 L/2]  Multiplication=Matrix(K*u)
  Mux : Mux  Inputs=2
  Radians to Degrees : simulink_extras/Transformations/Radians to Degrees
  Radians to Degrees1 : simulink_extras/Transformations/Radians to Degrees
  wl (deg/s) : Outport  VectorParamsAs1DForOutWhenUnconnected=off
  wr (deg/s) : Outport  Port=2  VectorParamsAs1DForOutWhenUnconnected=off
  wires:
  " Gain"/1 -> Demux/1
  Matrix multiplication/1 -> " Gain"/1
  v(cm/s)/1 -> Mux/1
  Mux/1 -> Matrix multiplication/1
  Demux/1 -> Radians to Degrees/1
  Demux/2 -> Radians to Degrees1/1
  w(deg/s)/1 -> Degrees to Radians/1
  Radians to Degrees/1 -> wl (deg/s)/1
  Radians to Degrees1/1 -> wr (deg/s)/1
  Degrees to Radians/1 -> Mux/2

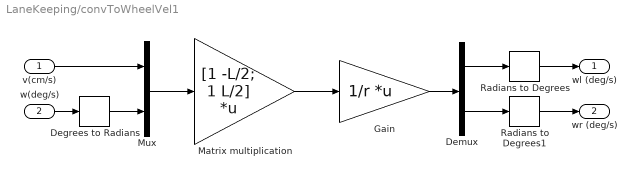
== system LaneKeeping/convToWheelVel1 ==
  v(cm/s) : Inport
  w(deg/s) : Inport  Port=2
  " Gain" : Gain  Gain=1/r  Multiplication=Matrix(K*u)
  Degrees to Radians : simulink_extras/Transformations/Degrees to Radians
  Demux : Demux  Outputs=2
  Matrix multiplication : Gain  Gain=[1 -L/2; 1 L/2]  Multiplication=Matrix(K*u)
  Mux : Mux  Inputs=2
  Radians to Degrees : simulink_extras/Transformations/Radians to Degrees
  Radians to Degrees1 : simulink_extras/Transformations/Radians to Degrees
  wl (deg/s) : Outport  VectorParamsAs1DForOutWhenUnconnected=off
  wr (deg/s) : Outport  Port=2  VectorParamsAs1DForOutWhenUnconnected=off
  wires:
  " Gain"/1 -> Demux/1
  Matrix multiplication/1 -> " Gain"/1
  v(cm/s)/1 -> Mux/1
  Mux/1 -> Matrix multiplication/1
  Demux/1 -> Radians to Degrees/1
  Demux/2 -> Radians to Degrees1/1
  w(deg/s)/1 -> Degrees to Radians/1
  Radians to Degrees/1 -> wl (deg/s)/1
  Radians to Degrees1/1 -> wr (deg/s)/1
  Degrees to Radians/1 -> Mux/2

== matlab function LaneKeeping/Individua linea centrale/mid_point2 ==
  data: u input; y output
function y = fcn(u)

y = int32(u(1)+u(2))/2;

== matlab function LaneKeeping/Individua linea centrale/mid_point3 ==
  data: u input; y output
function y = fcn(u)

y = int32(u(1)+u(2))/2;

== stateflow chart LaneKeeping/Chart ==
  state GoRight
    entry: v = 2
    w = -8
  state GoLeft
    entry: v = 2
    w = 8
  state StraightOn
    entry: v = 8
    w = 0
  StraightOn -> GoRight [order 2] : [distanza < -eps]
  GoRight -> StraightOn : [distanza >= -eps]
  StraightOn -> GoLeft [order 1] : [distanza > eps]
  GoLeft -> StraightOn : [distanza <= eps]
  (default) -> StraightOn
  data: distanza input; v output; w output; eps constant double =5

== stateflow chart LaneKeeping/Chart1 ==
  state GoRight
    entry: v = 2
    w = -8
  state GoLeft
    entry: v = 2
    w = 8
  state StraightOn
    entry: v = 8
    w = 0
  StraightOn -> GoRight [order 2] : [distanza < -eps]
  GoRight -> StraightOn : [distanza >= -eps]
  StraightOn -> GoLeft [order 1] : [distanza > eps]
  GoLeft -> StraightOn : [distanza <= eps]
  (default) -> StraightOn
  data: distanza input; v output; w output; eps constant double =5

== matlab function LaneKeeping/Individua linea centrale/mid_point ==
  data: u input; y output
function y = fcn(u)

y = int32(u(1)+u(2))/2;

== matlab function LaneKeeping/Individua linea centrale/mid_point1 ==
  data: u input; y output
function y = fcn(u)

y = int32(u(1)+u(2))/2;

== matlab function LaneKeeping/Individua linea centrale/MATLAB Function ==
  data: matrice input; risultato output size=[1 1 1 1]
function risultato = calcolaMatrice(matrice)

    % Verifica delle dimensioni della matrice di input
    assert(isequal(size(matrice), [2, 4]), 'La matrice deve essere di dimensioni 2x4.');
 
    % Calcola la media dei valori tra la 1x1 e la 2x1
    risultato = [mean(matrice(:, 1))];
 
    % Assegna il valore 1 alla posizione 1x2
    risultato = [risultato 1];
 
    % Calcola la media dei valori tra la 1x3 e la 2x3
    risultato = [risultato mean(matrice(:, 3))];
 
    % Assegna il valore 239 alla posizione 1x4
    risultato = [risultato 239];
